simulink model "lyskawaProject_si_rs"  (R2023b)
settings: Solver=VariableStepAuto  StartTime=startTime  StopTime=stopTime  MaxStep=maxStepSize  RelTol=1e-3
values from neighbouring files (symbols this model uses):
  dTk = 0    [lyskawaProject.m]    (also in nieliniowe.m; rStanu.m; transmitancje.m)
  dTz = 1    [lyskawaProject.m]    (also in nieliniowe.m = 0; rStanu.m = 2; transmitancje.m = 2)
  M1 = [(-cp*ro*fp0-K1-Kp)/Cvw, Kp/Cvw;(cp*ro*fp0+Kp)/Cvp, (-cp*ro*fp0-Kp-K2)/Cvp]    [lyskawaProject.m]
  M2 = [K1/Cvw, (cp*ro*fp0)/Cvw;K2/Cvp, 0]    [lyskawaProject.m]
  M3 = [1,0;0,1]    [lyskawaProject.m]
  M4 = [0,0 ; 0,0]    [lyskawaProject.m]
  t0 = 10    [lyskawaProject.m]    (also in nieliniowe.m = 100; rStanu.m = 100; test2.m; transmitancje.m = 100)
  Tk0 = TkN    (= 35)    [lyskawaProject.m]    (also in nieliniowe.m = vTk0(3); rStanu.m = vTk0(3); transmitancje.m = vTk0(3))
  Tz0 = TzN    (= -20)    [lyskawaProject.m]    (also in nieliniowe.m = vTz0(3); rStanu.m = vTz0(3); transmitancje.m = vTz0(3))
  x0 = -inv(M1)*M2*u    [lyskawaProject.m]
settings Model: Creator=aleklyskawa  LastModifiedBy=aleklyskawa

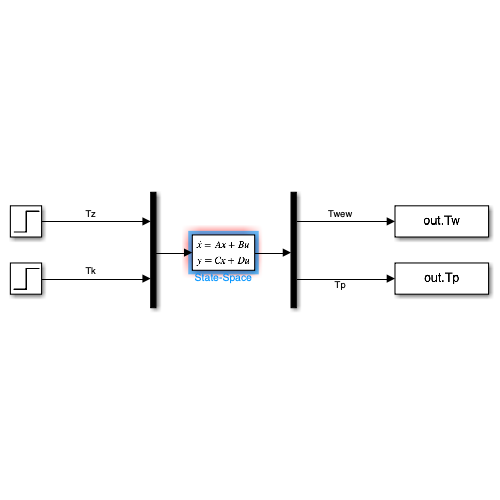
[thumbnail: Simulink's stored preview of the top-level diagram]
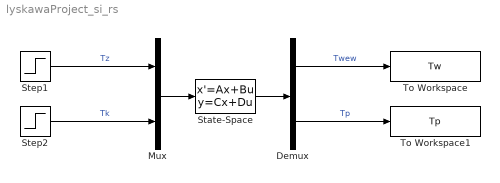
== system lyskawaProject_si_rs ==
  Demux : Demux  Outputs=2
  Mux : Mux  Inputs=2
  State-Space : StateSpace  A=M1  B=M2  C=M3  D=M4  InitialCondition=x0
  Step1 : Step  Time=t0  Before=Tz0  After=Tz0 + dTz  SampleTime=0
  Step2 : Step  Time=t0  Before=Tk0  After=Tk0+dTk  SampleTime=0
  To Workspace : ToWorkspace  VariableName=Tw  SampleTime=-1
  To Workspace1 : ToWorkspace  VariableName=Tp  SampleTime=-1
  wires:
  State-Space/1 -> Demux/1
  Mux/1 -> State-Space/1
  Demux/1 -> To Workspace/1  "Twew"
  Demux/2 -> To Workspace1/1  "Tp"
  Step1/1 -> Mux/1  "Tz"
  Step2/1 -> Mux/2  "Tk"
